simulink model "demo3"  (Simulink 4.00)
settings: Solver=ode45  StartTime=0.0  StopTime=10.0  RelTol=1e-3
undefined symbols (not defined in the file or in its folder): p560, perturb
libraries: roblocks x4, simulink3 x1
settings Model: Creator=pic  LastModifiedBy=pic  LimitDataPoints=off  ExtModeTrigMode=oneshot  ExtModeArmWhenConnect=off  BlockReductionOpt=off

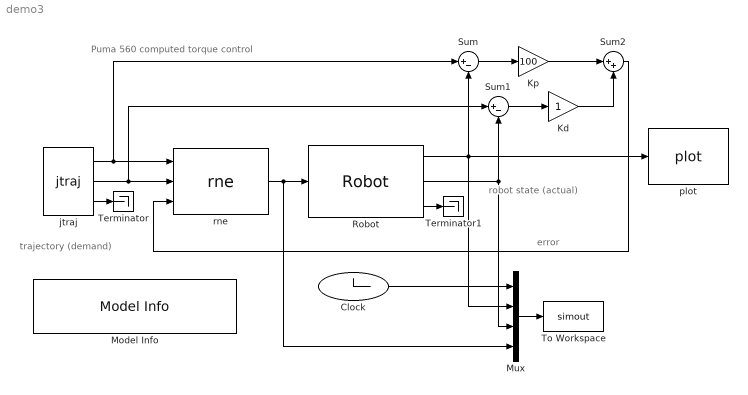
== system demo3 ==
  note: Puma 560 computed torque control
  note: trajectory
      | (demand)
  note: robot state
      | (actual)
  note: error
  Clock : Clock
      settings: Decimation=10
  Kd : Gain  Gain=1  Multiplication=Element-wise(K.*u)  SaturateOnIntegerOverflow=on
  Kp : Gain  Gain=100  Multiplication=Element-wise(K.*u)  SaturateOnIntegerOverflow=on
  Model Info : simulink3/Signals & Systems/Model Info  InitialBlockCM=none  BlockCM=none  Frame=on  DisplayStringWithTags=|  HorizontalTextAlignment=Left  LeftAlignmentValue=0.02  SourceBlockDiagram=demo3  TagMaxNumber=20
      | Puma560 computed torque control
      | %<Creator>
      | %<LastModificationDate>
  Mux : Mux  Inputs=4
  Robot : roblocks/Robot  robot=p560  q0=[0 0 0 0 0 0]
  Sum : Sum  Inputs=|+-  SaturateOnIntegerOverflow=on
  Sum1 : Sum  Inputs=|+-  SaturateOnIntegerOverflow=on
  Sum2 : Sum  Inputs=|++  SaturateOnIntegerOverflow=on
  Terminator : Terminator
  Terminator1 : Terminator
  To Workspace : ToWorkspace  VariableName=simout  SampleTime=-1  SaveFormat=Array
  jtraj : roblocks/jtraj  q0=[0 0 0 0 0 0]  qf=[pi/4 pi/2 -pi/2 0 0 0]  tmax=10
  plot : roblocks/plot  robot=p560
  rne : roblocks/rne  robot=perturb(p560)  grav=[0 0 9.81]
  wires:
  Sum/1 -> Kp/1
  Kp/1 -> Sum2/1
  Robot/1 -> plot/1, Mux/2, Sum/2
  Robot/2 -> Mux/3, Sum1/2
  Sum2/1 -> rne/3
  rne/1 -> Robot/1, Mux/4
  jtraj/1 -> Sum/1, rne/1
  jtraj/2 -> rne/2, Sum1/1
  Mux/1 -> To Workspace/1
  Clock/1 -> Mux/1
  Sum1/1 -> Kd/1
  Kd/1 -> Sum2/2
  jtraj/3 -> Terminator/1
  Robot/3 -> Terminator1/1
